simulink model "vrmaglev"  (Simulink 7.4)
settings: Solver=ode5  SolverMode=SingleTasking  StartTime=0.0  StopTime=Inf  FixedStep=1e-3  MaxStep=0.001  RelTol=1e-3  AbsTol=1e-5
PreLoadFcn:
  | Ts=1e-3;
libraries: vrlib x2, simulink x1
Description:
  | Magnetic Levitation Model
  | 
  | vrmaglev is an example showing the interaction between dynamic models in Simulink(R)
  | and virtual worlds. The Simulink model represents the HUMUSOFT(R) CE152 Magnetic Levitation
  | educational / presentation scale model. (http://www.humusoft.com/link/models)
  | 
  | The plant model is controlled by a PID controller with feed forward to cope with the nonlinearity
  | of the magnetic levitation system.
  | 
  | The position of the ball responds to the changing value of the setpoint. You can observe
  | this change not only in the Scope window, but also in a viewer window displaying
  | the virtual world. Note that the position of the ball represents the real dynamics of the system.
  | If you switch the VRML viewer to the Camera 3 viewpoint, you can observe and control the ball easier.
  | 
  | There are two possible methods of setting the ball position setpoint - using a Signal Generator
  | and visually by clicking at a desired position in the virtual reality scene.
  | 
  | In the virtual scene, a VRML sensor is defined. If you click in the space between the magnetic coil
  | and the bottom plate, VRML sensor is updated and its value is read into Simulink model using the
  | VR Sensor Reader block. The data connection is accomplished using an S-function (vrextin).
  | Look under mask of the VR Sensor Reader to see more details on how to read values
  | from virtual scenes programmatically.
settings Model: Creator=Sehnal  LastModifiedBy=miro  CovMetricSettings=d  ExtModeTrigDuration=5000  ExtModeTrigLevel=0.500000  BufferReuse=off
settings DataIOCC: LimitDataPoints=off  SaveOutput=off  SaveTime=off  SignalLoggingName=logsOut
settings OptimizationCC: BlockReduction=off  BooleanDataType=off  InlineInvariantSignals=on  OptimizeBlockIOStorage=off  BufferReuse=off  ExpressionFolding=off  LocalBlockOutputs=off  InitFltsAndDblsToZero=on
settings DebuggingCC: CheckExecutionContextPreStartOutputMsg=on  CheckExecutionContextRuntimeOutputMsg=on  SignalResolutionControl=TryResolveAllWithWarning  SolverPrmCheckMsg=none  MultiTaskDSMMsg=warning  MultiTaskCondExecSysMsg=none  StrictBusMsg=None
settings HardwareCC: TargetUnknown=on
settings ModelReferenceCC: UpdateModelReferenceTargets=IfOutOfDate
settings RTWCC: RetainRTWFile=on  IncludeERTFirstTime=on
settings GRTTargetCC: TargetFcnLib=ansi_tfl_tmw.mat

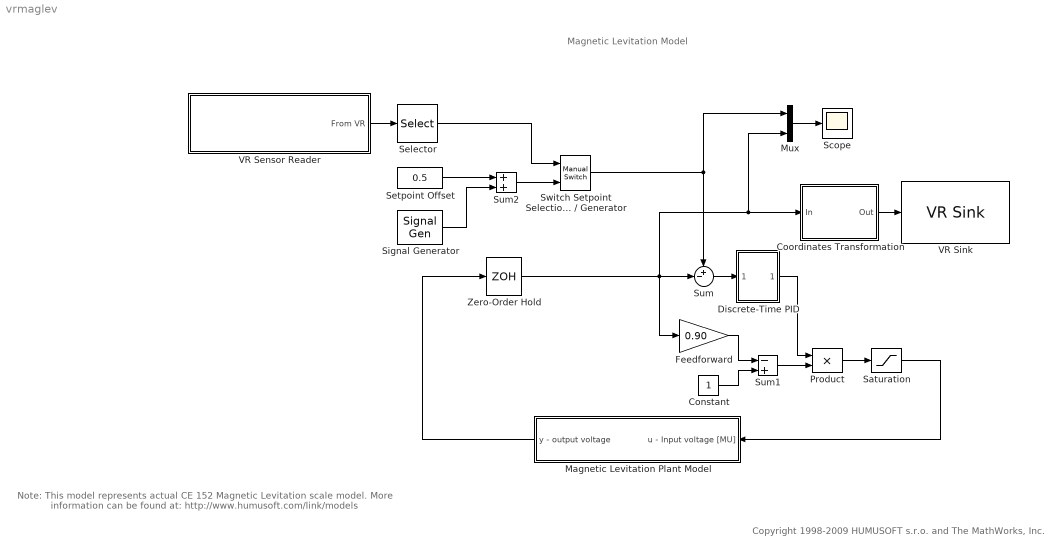
== system vrmaglev ==
  note: Magnetic Levitation Model
  note: Note:
      | This model represents actual CE 152 Magnetic Levitation scale model. More information can be found at:
      | http://www.humusoft.com/link/models
  note: Copyright 1998-2009 HUMUSOFT s.r.o. and The MathWorks, Inc.
  Constant : Constant  OutDataType=sfix(16)  OutScaling=2^0
  Coordinates Transformation : Subsystem
  Discrete-Time PID : Subsystem  mask(PID){Kp=1, Ki=10, Kd=0.03, Ts=Ts}
      mask prompts: Ts "Sample time:"
      mask help: Discrete-time PID controller with limited integrator
      mask Display: disp('PID');
  Feedforward : Gain  Gain=0.90  ParameterDataType=sfix(16)  ParameterScaling=2^0  OutDataType=sfix(16)  OutScaling=2^0  SaturateOnIntegerOverflow=on  OutDataTypeStr=Inherit: Same as input  ParamDataTypeStr=Inherit: Same as input
  Magnetic Levitation Plant Model : Subsystem
  Mux : Mux  Inputs=2
  Product : Product  OutDataType=sfix(16)  OutScaling=2^0  SaturateOnIntegerOverflow=on  InputSameDT=on  OutDataTypeStr=Inherit: Same as first input
  Saturation : Saturate  UpperLimit=1  LowerLimit=0  ZeroCross=off  OutDataType=sfix(16)  OutScaling=2^0
  Scope : Scope
      settings: TimeRange=5  YMin=-0.0227122  YMax=1.027  DataFormat=Structure  MaxDataPoints=250  SampleInput=on  SampleTime=0.02
  Selector : Selector  InputPortWidth=3  IndexOptions=Index vector (dialog)  Indices=[2]  OutputSizes=1
  Setpoint Offset : Constant  Value=0.5  OutDataType=sfix(16)  OutScaling=2^0
  Signal Generator : SignalGenerator  WaveForm=square  Amplitude=0.1  Frequency=7  Units=rad/sec
  Sum : Sum  Inputs=+-|  OutDataType=sfix(16)  OutScaling=2^0  SaturateOnIntegerOverflow=on  InputSameDT=on  OutDataTypeStr=Inherit: Same as first input
  Sum1 : Sum  Inputs=-+  OutDataType=sfix(16)  OutScaling=2^0  SaturateOnIntegerOverflow=on  InputSameDT=on  OutDataTypeStr=Inherit: Same as first input
  Sum2 : Sum  OutDataType=sfix(16)  OutScaling=2^0  SaturateOnIntegerOverflow=on  InputSameDT=on  OutDataTypeStr=Inherit: Same as first input
  Switch Setpoint Selection Method Virtual Reality / Generator : simulink/Signal Routing/Manual Switch  SystemSampleTime=-1  sw=0  action=0  varsize=off
  VR Sensor Reader : Subsystem  mask(VR Sensor Reader){Ts=0.1, vr_world='maglev.wrl', vr_field='Grab_Sensor.translation_changed'}
      mask prompts: Ts "Sample time:"; vr_world "VRML world name:"; vr_field "VRML Node.Field name:"
      mask help: Read value from an exposed VRML field of a VRML scene (usually a VRML sensor output field).
      mask Display: image(imread('vrblockicon.png')); port_label('output', 1, vr_field);
  VR Sink : vrlib/VR Sink  InstantiateOnLoad=on  SampleTime=0.1  ViewEnable=on  RemoteChange=off  RemoteView=off  FieldsWritten=Ball.translation.3.1.double  WorldFileName=maglev.wrl  AutoView=on  VideoDimensions=[]  FigureProperties="{'Position', 'Name', 'Viewpoint', 'CameraBound', 'CameraDirection', 'CameraPosition', 'CameraUpVector', 'ZoomFactor', 'Antialiasing', 'Headlight', 'Lighting', 'NavPanel', 'StatusBar', 'ToolBar', 'Textures', 'Transparency', 'Wireframe', 'NavZones', 'NavMode', 'NavSpeed', 'Record2DCompressMethod', 'Record2DCompressQuality', 'Record2D', 'Record2DFileName', 'Record2DFPS'; [4.0000000000000000e+000  7.7000000000000000e+001  5.7600000000000000e+002  3.8000000000000000e+002], 'VR Magnetic Levitation Model', 'Camera 3', 'on', [-8.7932987404324714e-001 -4.5238500617408051e-001  1.4875072706995052e-001], [2.1054995483159640e+001  1.1038694313748776e+001 -1.9130532265516603e+001], [-4.2631905968288247e-001  8.8700260830278899e-001  1.7742162273844447e-001], [1.0000000000000000e+000], 'off', 'off', 'on', 'halfbar', 'off', 'on', 'on', 'on', 'off', 'off', 'examine', 'normal', 'auto', [7.5000000000000000e+001], 'off', '%f_anim_%n.avi', [1.5000000000000000e+001]}"
  Zero-Order Hold : ZeroOrderHold  SampleTime=Ts
  wires:
  Constant/1 -> Sum1/2
  Sum1/1 -> Product/2
  Feedforward/1 -> Sum1/1
  Sum/1 -> Discrete-Time PID/1(in_1)
  Discrete-Time PID/1(out_1) -> Product/1
  Switch Setpoint Selection Method Virtual Reality / Generator/1 -> Sum/1, Mux/1
  Zero-Order Hold/1 -> Sum/2, Feedforward/1, Coordinates Transformation/1(In), Mux/2
  Mux/1 -> Scope/1
  Product/1 -> Saturation/1
  Magnetic Levitation Plant Model/1(y - output voltage) -> Zero-Order Hold/1
  Coordinates Transformation/1(Out) -> VR Sink/1
  Saturation/1 -> Magnetic Levitation Plant Model/1(u - Input voltage [MU])
  Sum2/1 -> Switch Setpoint Selection Method Virtual Reality / Generator/2
  Signal Generator/1 -> Sum2/2
  Setpoint Offset/1 -> Sum2/1
  VR Sensor Reader/1(From VR) -> Selector/1
  Selector/1 -> Switch Setpoint Selection Method Virtual Reality / Generator/1

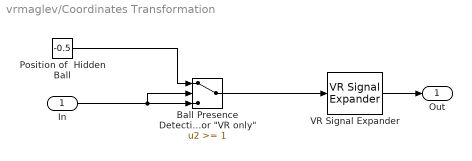
== system vrmaglev/Coordinates Transformation ==
  In : Inport  OutDataType=sfix(16)  OutScaling=2^0
  "Ball Presence Detection Value > Threshold = Ball Not Present 1 for \"VR only\"" : Switch  Threshold=1  OutDataType=sfix(16)  OutScaling=2^0  InputSameDT=on
  Position of  Hidden Ball : Constant  Value=-0.5  OutDataType=sfix(16)  OutScaling=2^0
  VR Signal Expander : vrlib/VR Signal Expander  SystemSampleTime=-1  outwidth=3  outidx=[2]
  Out : Outport  OutDataType=sfix(16)  OutScaling=2^0
  wires:
  Position of  Hidden Ball/1 -> "Ball Presence Detection Value > Threshold = Ball Not Present 1 for \"VR only\""/1
  In/1 -> "Ball Presence Detection Value > Threshold = Ball Not Present 1 for \"VR only\""/3, "Ball Presence Detection Value > Threshold = Ball Not Present 1 for \"VR only\""/2
  "Ball Presence Detection Value > Threshold = Ball Not Present 1 for \"VR only\""/1 -> VR Signal Expander/1
  VR Signal Expander/1 -> Out/1

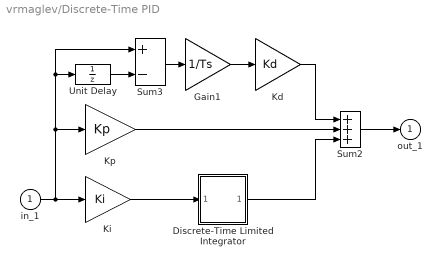
== system vrmaglev/Discrete-Time PID ==
  in_1 : Inport  OutDataType=sfix(16)  OutScaling=2^0
  Discrete-Time Limited Integrator : Subsystem  mask(Discrete-Time Limited Integrator.){@1=0, @2=2, @3=0, @4=Ts}
      mask prompts: @1 "Lower bound:"; @2 "Upper bound:"; @3 "Initial condition:"; @4 "Sampling Time:"
      mask help: Discrete-Time Limited Integrator.
      mask init:
      | lower_limit=@1;upper_limit=@2;X0=@3;Ts=@4;
      mask Help: Discrete-Time Limited Integrator. Unmask to see details.
      mask Display: plot(-1,-0.2,3.5,1.2,[0,1,2,2.9],[0,0,1,1],[0,1],[0.5,0.5], [.5,.5], [.8,.6], [.05,.35,.05,.35],[.4,.4,.2,.2], [.45,.65],[.3,.3], [.9,.9],[.2,.4]);
  Gain1 : Gain  Gain=1/Ts  ParameterDataType=sfix(16)  ParameterScaling=2^0  OutDataType=sfix(16)  OutScaling=2^0  SaturateOnIntegerOverflow=on  OutDataTypeStr=Inherit: Same as input  ParamDataTypeStr=Inherit: Same as input
  Kd : Gain  Gain=Kd  ParameterDataType=sfix(16)  ParameterScaling=2^0  OutDataType=sfix(16)  OutScaling=2^0  SaturateOnIntegerOverflow=on  OutDataTypeStr=Inherit: Same as input  ParamDataTypeStr=Inherit: Same as input
  Ki : Gain  Gain=Ki  ParameterDataType=sfix(16)  ParameterScaling=2^0  OutDataType=sfix(16)  OutScaling=2^0  SaturateOnIntegerOverflow=on  OutDataTypeStr=Inherit: Same as input  ParamDataTypeStr=Inherit: Same as input
  Kp : Gain  Gain=Kp  ParameterDataType=sfix(16)  ParameterScaling=2^0  OutDataType=sfix(16)  OutScaling=2^0  SaturateOnIntegerOverflow=on  OutDataTypeStr=Inherit: Same as input  ParamDataTypeStr=Inherit: Same as input
  Sum2 : Sum  Inputs=+++  OutDataType=sfix(16)  OutScaling=2^0  SaturateOnIntegerOverflow=on  InputSameDT=on  OutDataTypeStr=Inherit: Same as first input
  Sum3 : Sum  Inputs=+-  OutDataType=sfix(16)  OutScaling=2^0  SaturateOnIntegerOverflow=on  InputSameDT=on  OutDataTypeStr=Inherit: Same as first input
  Unit Delay : UnitDelay  SampleTime=Ts
  out_1 : Outport  OutDataType=sfix(16)  OutScaling=2^0  InitialOutput=0
  wires:
  Unit Delay/1 -> Sum3/2
  Kd/1 -> Sum2/1
  Kp/1 -> Sum2/2
  Sum2/1 -> out_1/1
  Sum3/1 -> Gain1/1
  Gain1/1 -> Kd/1
  in_1/1 -> Ki/1, Sum3/1, Unit Delay/1, Kp/1
  Ki/1 -> Discrete-Time Limited Integrator/1(in_1)
  Discrete-Time Limited Integrator/1(out_1) -> Sum2/3

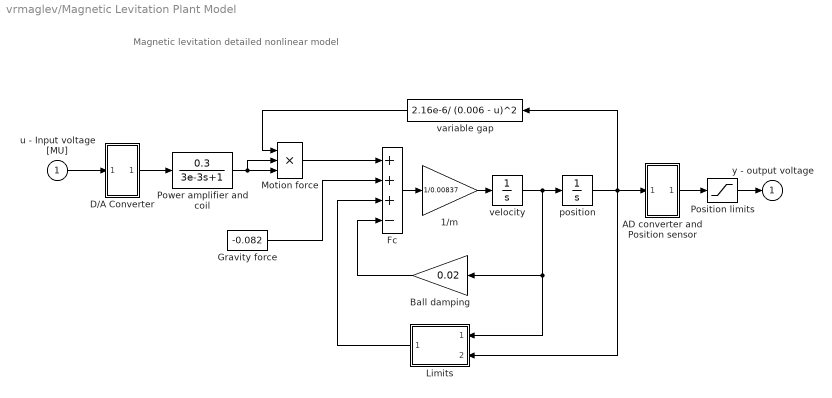
== system vrmaglev/Magnetic Levitation Plant Model ==
  note: Magnetic levitation
      | detailed nonlinear model
  u - Input voltage [MU] : Inport  OutDataType=sfix(16)  OutScaling=2^0
  1/m : Gain  Gain=1/0.00837  ParameterDataType=sfix(16)  ParameterScaling=2^0  OutDataType=sfix(16)  OutScaling=2^0  SaturateOnIntegerOverflow=on  OutDataTypeStr=Inherit: Same as input  ParamDataTypeStr=Inherit: Same as input
  AD converter and Position sensor : Subsystem
      mask Display: disp('A/D')
  Ball damping : Gain  Gain=0.02  ParameterDataType=sfix(16)  ParameterScaling=2^0  OutDataType=sfix(16)  OutScaling=2^0  SaturateOnIntegerOverflow=on  OutDataTypeStr=Inherit: Same as input  ParamDataTypeStr=Inherit: Same as input
  D/A Converter : Subsystem
      mask Display: disp('D/A')
  Fc : Sum  Inputs=+++-  OutDataType=sfix(16)  OutScaling=2^0  SaturateOnIntegerOverflow=on  InputSameDT=on  OutDataTypeStr=Inherit: Same as first input
  Gravity force : Constant  Value=-0.082  OutDataType=sfix(16)  OutScaling=2^0
  Limits : Subsystem
      mask Display: disp('LIMIT')
  Motion force : Product  Inputs=3  OutDataType=sfix(16)  OutScaling=2^0  SaturateOnIntegerOverflow=on  InputSameDT=on  OutDataTypeStr=Inherit: Same as first input
  Position limits : Saturate  UpperLimit=0.998  LowerLimit=0  ZeroCross=off  OutDataType=sfix(16)  OutScaling=2^0
  Power amplifier and coil : TransferFcn  Numerator=[0.3]  Denominator=[3e-3 1]
  position : Integrator  LimitOutput=on  UpperSaturationLimit=0.005  LowerSaturationLimit=0  ZeroCross=off
  variable gap : Fcn  Expr=2.16e-6/ (0.006 - u)^2
  velocity : Integrator  UpperSaturationLimit=Inf  LowerSaturationLimit=-Inf  ZeroCross=off
  y - output voltage : Outport  OutDataType=sfix(16)  OutScaling=2^0
  wires:
  velocity/1 -> Ball damping/1, Limits/1(velocity), position/1
  Ball damping/1 -> Fc/4
  variable gap/1 -> Motion force/1
  1/m/1 -> velocity/1
  Fc/1 -> 1/m/1
  Motion force/1 -> Fc/1
  Gravity force/1 -> Fc/2
  D/A Converter/1(out_1) -> Power amplifier and coil/1
  u - Input voltage [MU]/1 -> D/A Converter/1(in_1)
  AD converter and Position sensor/1(out_1) -> Position limits/1
  position/1 -> Limits/2(position), variable gap/1, AD converter and Position sensor/1(in_1)
  Limits/1(force) -> Fc/3
  Power amplifier and coil/1 -> Motion force/3, Motion force/2
  Position limits/1 -> y - output voltage/1

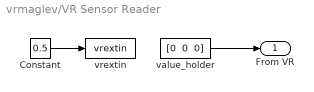
== system vrmaglev/VR Sensor Reader ==
  Constant : Constant  Value=0.5  OutDataType=sfix(16)  OutScaling=2^0
  value_holder : Constant  Value="[0  0  0]"  OutDataType=sfix(16)  OutScaling=2^0
  vrextin : S-Function  FunctionName=vrextin  Parameters=Ts, 'maglev.wrl', 'Grab_Sensor.translation_changed'  EnableBusSupport=off
  From VR : Outport  OutDataType=sfix(16)  OutScaling=2^0
  wires:
  value_holder/1 -> From VR/1
  Constant/1 -> vrextin/1

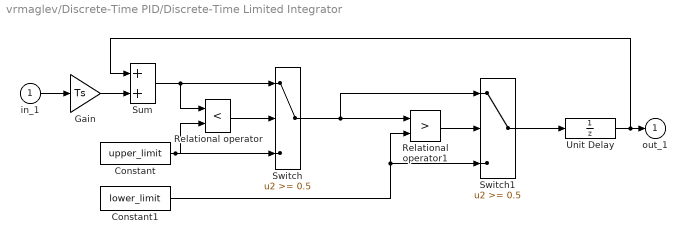
== system vrmaglev/Discrete-Time PID/Discrete-Time Limited Integrator ==
  in_1 : Inport  OutDataType=sfix(16)  OutScaling=2^0
  Constant : Constant  Value=upper_limit  OutDataType=sfix(16)  OutScaling=2^0
  Constant1 : Constant  Value=lower_limit  OutDataType=sfix(16)  OutScaling=2^0
  Gain : Gain  Gain=Ts  ParameterDataType=sfix(16)  ParameterScaling=2^0  OutDataType=sfix(16)  OutScaling=2^0  SaturateOnIntegerOverflow=on  OutDataTypeStr=Inherit: Same as input  ParamDataTypeStr=Inherit: Same as input
  Relational operator : RelationalOperator  Operator=<  InputSameDT=on
  Relational operator1 : RelationalOperator  Operator=>  InputSameDT=on
  Sum : Sum  OutDataType=sfix(16)  OutScaling=2^0  SaturateOnIntegerOverflow=on  InputSameDT=on  OutDataTypeStr=Inherit: Same as first input
  Switch : Switch  Threshold=0.5  OutDataType=sfix(16)  OutScaling=2^0  InputSameDT=on
  Switch1 : Switch  Threshold=0.5  OutDataType=sfix(16)  OutScaling=2^0  InputSameDT=on
  Unit Delay : UnitDelay  X0=X0  SampleTime=Ts
  out_1 : Outport  OutDataType=sfix(16)  OutScaling=2^0  InitialOutput=0
  wires:
  Unit Delay/1 -> out_1/1, Sum/1
  Switch1/1 -> Unit Delay/1
  Constant1/1 -> Relational operator1/2, Switch1/3
  Relational operator1/1 -> Switch1/2
  Switch/1 -> Relational operator1/1, Switch1/1
  Constant/1 -> Switch/3, Relational operator/2
  Gain/1 -> Sum/2
  Sum/1 -> Switch/1, Relational operator/1
  Relational operator/1 -> Switch/2
  in_1/1 -> Gain/1

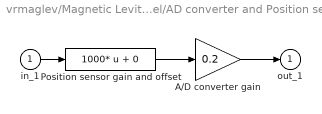
== system vrmaglev/Magnetic Levitation Plant Model/AD converter and Position sensor ==
  in_1 : Inport  OutDataType=sfix(16)  OutScaling=2^0
  A/D converter gain : Gain  Gain=0.2  ParameterDataType=sfix(16)  ParameterScaling=2^0  OutDataType=sfix(16)  OutScaling=2^0  SaturateOnIntegerOverflow=on  OutDataTypeStr=Inherit: Same as input  ParamDataTypeStr=Inherit: Same as input
  Position sensor gain and offset : Fcn  Expr=1000* u + 0
  out_1 : Outport  OutDataType=sfix(16)  OutScaling=2^0
  wires:
  in_1/1 -> Position sensor gain and offset/1
  Position sensor gain and offset/1 -> A/D converter gain/1
  A/D converter gain/1 -> out_1/1

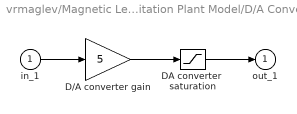
== system vrmaglev/Magnetic Levitation Plant Model/D/A Converter ==
  in_1 : Inport  OutDataType=sfix(16)  OutScaling=2^0
  D/A converter gain : Gain  Gain=5  ParameterDataType=sfix(16)  ParameterScaling=2^0  OutDataType=sfix(16)  OutScaling=2^0  SaturateOnIntegerOverflow=on  OutDataTypeStr=Inherit: Same as input  ParamDataTypeStr=Inherit: Same as input
  DA converter  saturation : Saturate  UpperLimit=5  LowerLimit=-5  ZeroCross=off  OutDataType=sfix(16)  OutScaling=2^0
  out_1 : Outport  OutDataType=sfix(16)  OutScaling=2^0
  wires:
  in_1/1 -> D/A converter gain/1
  DA converter  saturation/1 -> out_1/1
  D/A converter gain/1 -> DA converter  saturation/1

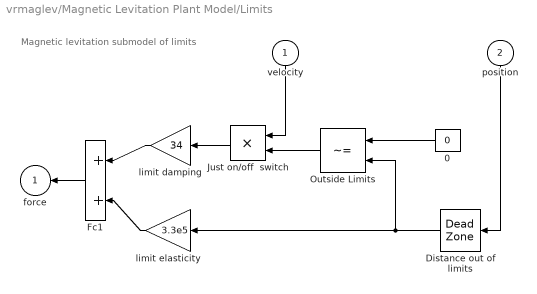
== system vrmaglev/Magnetic Levitation Plant Model/Limits ==
  note: Magnetic levitation
      | submodel of limits
  velocity : Inport  OutDataType=sfix(16)  OutScaling=2^0
  position : Inport  Port=2  OutDataType=sfix(16)  OutScaling=2^0
  0 : Constant  Value=0  OutDataType=sfix(16)  OutScaling=2^0
  Distance out of limits : DeadZone  LowerValue=0  UpperValue=0.005  ZeroCross=off  SaturateOnIntegerOverflow=on
  Fc1 : Sum  OutDataType=sfix(16)  OutScaling=2^0  SaturateOnIntegerOverflow=on  InputSameDT=on  OutDataTypeStr=Inherit: Same as first input
  "Just on/off  switch " : Product  OutDataType=sfix(16)  OutScaling=2^0  SaturateOnIntegerOverflow=on  InputSameDT=on  OutDataTypeStr=Inherit: Same as first input
  Outside Limits : RelationalOperator  Operator=~=  InputSameDT=on
  limit damping : Gain  Gain=34  ParameterDataType=sfix(16)  ParameterScaling=2^0  OutDataType=sfix(16)  OutScaling=2^0  SaturateOnIntegerOverflow=on  OutDataTypeStr=Inherit: Same as input  ParamDataTypeStr=Inherit: Same as input
  limit elasticity : Gain  Gain=3.3e5  ParameterDataType=sfix(16)  ParameterScaling=2^0  OutDataType=sfix(16)  OutScaling=2^0  SaturateOnIntegerOverflow=on  OutDataTypeStr=Inherit: Same as input  ParamDataTypeStr=Inherit: Same as input
  force : Outport  OutDataType=sfix(16)  OutScaling=2^0
  wires:
  Distance out of limits/1 -> Outside Limits/2, limit elasticity/1
  limit damping/1 -> Fc1/1
  limit elasticity/1 -> Fc1/2
  Outside Limits/1 -> "Just on/off  switch "/2
  0/1 -> Outside Limits/1
  "Just on/off  switch "/1 -> limit damping/1
  velocity/1 -> "Just on/off  switch "/1
  Fc1/1 -> force/1
  position/1 -> Distance out of limits/1
